simulink model "pushpull"  (R2023b)
settings: Solver=VariableStepAuto  StartTime=0.0  StopTime=2  RelTol=1e-3
libraries: spsDiodeLib x2, spsIGBTLib x2, spsVoltageMeasurementLib x2, spsDCVoltageSourceLib x1, spsMultiWindingTransformerLib x1, spspowerguiLib x1
settings Model: Creator=Akaashdeep B  LastModifiedBy=Akaashdeep B

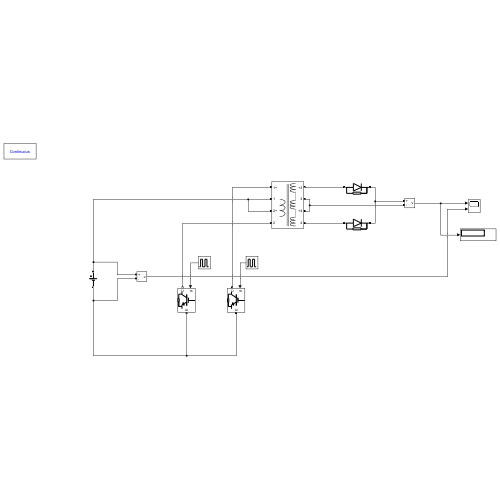
[thumbnail: Simulink's stored preview of the top-level diagram]
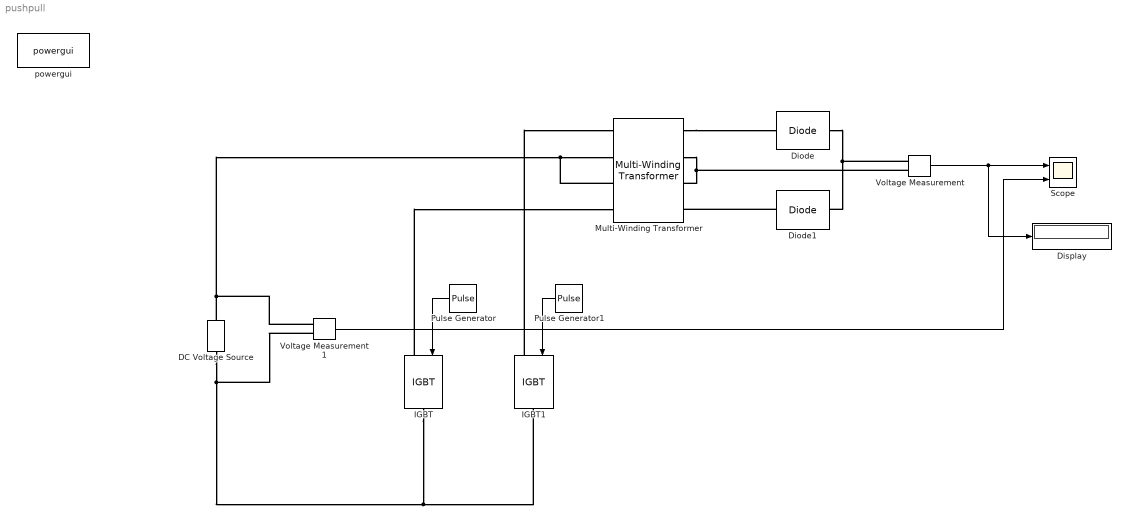
== system pushpull ==
  DC Voltage Source : spsDCVoltageSourceLib/DC Voltage Source  Amplitude=100  Measurements=None
  Diode : spsDiodeLib/Diode  Ron=0.001  Lon=0  Vf=0.8  IC=0  UseSnubber=0  Rs=500  Cs=250e-9  Measurements=off
  Diode1 : spsDiodeLib/Diode  Ron=0.001  Lon=0  Vf=0.8  IC=0  UseSnubber=0  Rs=500  Cs=250e-9  Measurements=off
  Display : Display
  IGBT : spsIGBTLib/IGBT  Ron=0.001  Lon=0  Vf=1  Tf=1e-6  Tt=2e-6  IC=0  Rs=1e5  Cs=inf  Measurements=off
  IGBT1 : spsIGBTLib/IGBT  Ron=0.001  Lon=0  Vf=1  Tf=1e-6  Tt=2e-6  IC=0  Rs=1e5  Cs=inf  Measurements=off
  Multi-Winding Transformer : spsMultiWindingTransformerLib/Multi-Winding Transformer  LeftWindings=2  RightWindings=2  TappedWindings=no taps  NumberOfTaps=2  SetSaturation=off  Hysteresis=off  DataFile='hysteresis.mat'  Measurements=None  UNITS=pu  NominalPower=[100 1000]  NominalVoltages=[ 100 100 25 25 ]  WindingResistances="[ 0.005  0.005  0.005  0.005]"  WindingInductances="[ 0.02  0.02  0.02  0.02 ]"  Rm=50  Lm=50  Saturation=[ 0,0 ; 0.0024,1.2 ; 1.0,1.52 ]  SpecifyInitialFlux=off  InitialFlux=0  BreakLoop=off  DiscreteSolver=Trapezoidal iterative  DataType=off  TransfoNumber=1
      settings: LibrarySourceBlock=|
      | sps_lib/Power Grid Elements/Multi-Winding
      | Transformer
  Pulse Generator : DiscretePulseGenerator  PulseType=Time based  Period=0.001  PulseWidth=50
  Pulse Generator1 : DiscretePulseGenerator  PulseType=Time based  Period=0.001  PulseWidth=50  PhaseDelay=0.0005
  Scope : Scope  NumInputPorts=2
  Voltage Measurement : spsVoltageMeasurementLib/Voltage Measurement  PhasorSimulation=off  OutputType=Complex  PSBequivalent=0
  Voltage Measurement1 : spsVoltageMeasurementLib/Voltage Measurement  PhasorSimulation=off  OutputType=Complex  PSBequivalent=0
  powergui : spspowerguiLib/powergui  Priority=1  SimulationMode=Continuous  SampleTime=50e-6  frequency=60  Iterations=50  frequencyindice=0  Pbase=100e6  ErrMax=1e-4  UnitsV=kV  UnitsW=MW  buscounter=0  FunctionMessages=off  echomessages=off  EnableUseOfTLC=off  CurrentSourceSwitches=off  DisableSnubberDevices=off  DisableRonSwitches=off  DisableVfSwitches=off  DisplayEquations=off  AutomaticDiscreteSolvers=off  SolverType=Tustin/Backward Euler (TBE)  Interpol=off  ExternalGateDelay=off  methode=off  Ts=100  x0status=blocks  SPID=on  SwTol=0  HookPort=off  NonlinearTolerance=1e-4  nMaxIteration=100  ContinueOnMaxIteration=off  RestoreLinks=warning  ResistiveCurrentMeasurement=off  Frange=[0:2:500]  Ylog=off  Xlog=on  ShowGrid=off  save=off  variable=ZData  structure=0  ZoomFFT=off  StartTime=0.0  cycles=1  DisplayStyle=1  fundamental=60  FreqAxis=off  MaxFrequency=1000  frequencyindicesteady=1  RmsSteady=1  display=off
  wires:
  Voltage Measurement/1 -> Display/1, Scope/1
  Voltage Measurement1/1 -> Scope/2
  Pulse Generator/1 -> IGBT/1
  Pulse Generator1/1 -> IGBT1/1
  connections:
  DC Voltage Source/RConn1 -- Voltage Measurement1/LConn1 -- Multi-Winding Transformer/LConn3 -- Multi-Winding Transformer/LConn2
  IGBT1/LConn1 -- Multi-Winding Transformer/LConn1
  IGBT/LConn1 -- Multi-Winding Transformer/LConn4
  DC Voltage Source/LConn1 -- Voltage Measurement1/LConn2 -- IGBT/RConn1 -- IGBT1/RConn1
  Multi-Winding Transformer/RConn1 -- Diode/LConn1
  Diode1/LConn1 -- Multi-Winding Transformer/RConn4
  Diode/RConn1 -- Voltage Measurement/LConn1 -- Diode1/RConn1
  Multi-Winding Transformer/RConn2 -- Voltage Measurement/LConn2 -- Multi-Winding Transformer/RConn3
